simulink model "RST"  (R2022b)
settings: Solver=FixedStepAuto  StartTime=0.0  StopTime=10  FixedStep=0.023  RelTol=1e-3
values from neighbouring files (symbols this model uses):
  G = tf(1,[0.1 1.1 1])    [RST.m]    (also in rst_1.m = tf(1,[Tao 1]); rst_2.m = 3/((s+3)*(s+9)); rst_incremental_1_orden.m = 3/((s+3)*(s+15)))
  T = sum(Qi)/sum(B_1)    [rst_1.m]    (also in rst_2.m; rst_incremental_1_orden.m = s0+s1+s2)
undefined symbols (not defined in the file or in its folder): dcgain
libraries: cstblocks x4
settings Model: Creator=omard  LastModifiedBy=omard

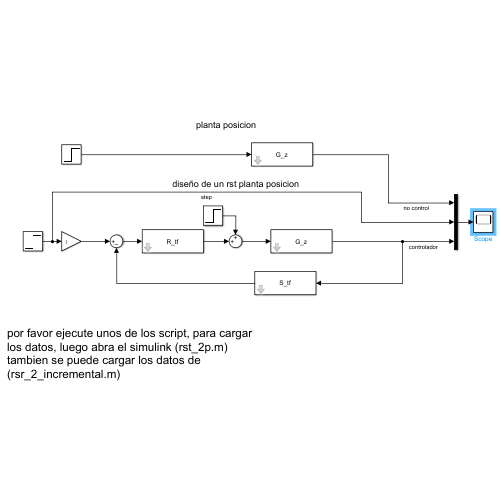
[thumbnail: Simulink's stored preview of the top-level diagram]
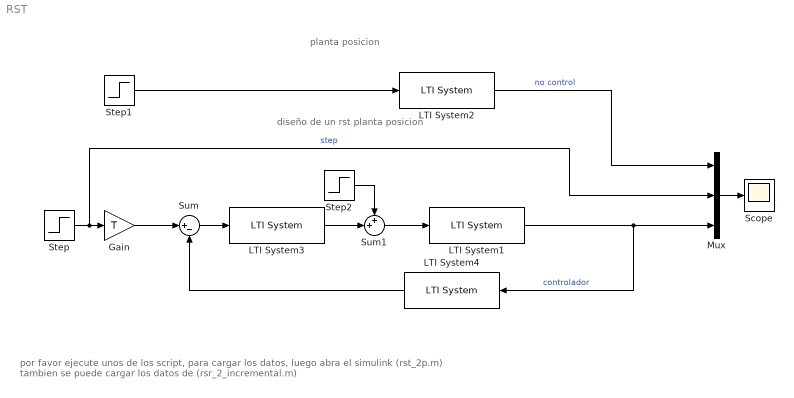
== system RST ==
  note: por favor ejecute unos de los script, para cargar los datos, luego abra el simulink (rst_2p.m) tambien se puede cargar los datos de (rsr_2_incremental.m)
  note: diseño de un rst planta posicion
  note: planta posicion
  Gain : Gain  Gain=T
  LTI System1 : cstblocks/LTI System  sys=G_z  IC=[]
  LTI System2 : cstblocks/LTI System  sys=G_z  IC=[]
  LTI System3 : cstblocks/LTI System  sys=R_tf  IC=[]
  LTI System4 : cstblocks/LTI System  sys=S_tf  IC=[]
  Mux : Mux  Inputs=3
  Scope : Scope
  Step : Step  After=dcgain(G)  SampleTime=0
  Step1 : Step  SampleTime=0
  Step2 : Step  Time=7  After=0.1  SampleTime=0
  Sum : Sum  Inputs=|+-
  Sum1 : Sum  Inputs=++|
  wires:
  Mux/1 -> Scope/1
  LTI System1/1 -> LTI System4/1, Mux/3  "controlador"
  LTI System2/1 -> Mux/1  "no control"
  Step1/1 -> LTI System2/1
  Sum/1 -> LTI System3/1
  Gain/1 -> Sum/1
  Step/1 -> Mux/2, Gain/1  "step"
  LTI System4/1 -> Sum/2
  Sum1/1 -> LTI System1/1
  LTI System3/1 -> Sum1/2
  Step2/1 -> Sum1/1
